simulink model "Equaliser"  (R2021b)
settings: Solver=VariableStepAuto  StartTime=0.0  StopTime=inf  RelTol=1e-3
model workspace (MAT data in the model file):
  D = Simulink.Parameter
  D.DataType = 'auto'
  D.Complexity = 'real'
  D.Dimensions = [0 0]
undefined symbols (not defined in the file): fdesignblkfcn, gcbh
libraries: dspfdesign x2, dspvision x1, dspobslib x1
settings Model: Creator=coren  LastModifiedBy=coren

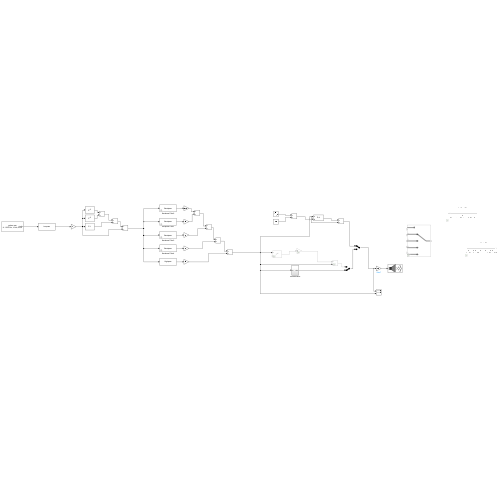
[thumbnail: Simulink's stored preview of the top-level diagram]
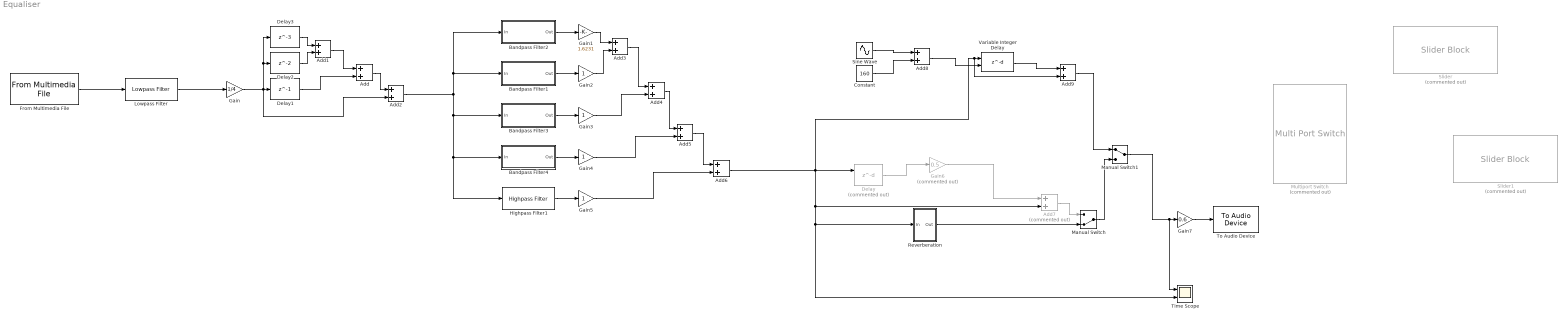
== system Equaliser ==
  Add{,1..6,8..9} (9 alike) : Sum
  Add7 : Sum  Commented=on
  Bandpass Filter1 : Subsystem  DialogController=fdesignblkfcn  InitFcn=fdesignblkfcn(gcbh, {'InitFcn'});  mask(Bandpass Filter){}
      mask help: Design a bandpass filter
      settings: CopyFcn=fdesignblkfcn(gcbh, {'CopyFcn'});
      mask Help: helpview(mapfilelocation('dsp'), 'dspbandpassfilter');
      mask Display: disp('Bandpass');
  Bandpass Filter2 : Subsystem  DialogController=fdesignblkfcn  InitFcn=fdesignblkfcn(gcbh, {'InitFcn'});  mask(Bandpass Filter){}
      mask help: Design a bandpass filter
      settings: CopyFcn=fdesignblkfcn(gcbh, {'CopyFcn'});
      mask Help: helpview(mapfilelocation('dsp'), 'dspbandpassfilter');
      mask Display: disp('Bandpass');
  Bandpass Filter3 : Subsystem  DialogController=fdesignblkfcn  InitFcn=fdesignblkfcn(gcbh, {'InitFcn'});  mask(Bandpass Filter){}
      mask help: Design a bandpass filter
      settings: CopyFcn=fdesignblkfcn(gcbh, {'CopyFcn'});
      mask Help: helpview(mapfilelocation('dsp'), 'dspbandpassfilter');
      mask Display: disp('Bandpass');
  Bandpass Filter4 : Subsystem  DialogController=fdesignblkfcn  InitFcn=fdesignblkfcn(gcbh, {'InitFcn'});  mask(Bandpass Filter){}
      mask help: Design a bandpass filter
      settings: CopyFcn=fdesignblkfcn(gcbh, {'CopyFcn'});
      mask Help: helpview(mapfilelocation('dsp'), 'dspbandpassfilter');
      mask Display: disp('Bandpass');
  Constant : Constant  Value=160
  Delay : Delay  Commented=on  DelayLengthSource=Input port  DelayLength=400  DelayLengthUpperLimit=5000  InputProcessing=Columns as channels (frame based)
      settings: InputPortMap=u0,p1
  Delay1 : Delay  DelayLength=1  DelayLengthUpperLimit=5000  InputProcessing=Columns as channels (frame based)
  Delay2 : Delay  DelayLengthUpperLimit=5000  InputProcessing=Columns as channels (frame based)
  Delay3 : Delay  DelayLength=3  DelayLengthUpperLimit=5000  InputProcessing=Columns as channels (frame based)
  From Multimedia File : dspvision/From Multimedia File  inputFilename=C:\Users\coren\Documents\MATLAB\Traitement Images et Son 3E105\Projet Son\guitare.wav  readRange=[1 Inf]  loop=on  numPlays=inf  outputStreams=Audio only  videoDataType=single  audioDataType=double  inheritSampleTime=on  userDefinedSampleTime=1/30  noAudioOutput=off  isIntensityVideo=off  fourcc=RGB  colorVideoFormat=Separate color signals  outputEOF=off  dataOrg=Column-major  audioFrameSize=1024  computeAudioFrameSize=off  outSamplingMode=Sample based
  Gain : Gain  Gain=1/4
  Gain1 : Gain  Gain=1.6231
  Gain{2..5} (4 alike) : Gain
  Gain6 : Gain  Commented=on  Gain=0.5
  Gain7 : Gain  Gain=0.6
  Highpass Filter1 : dspfdesign/Highpass Filter  FilterType=FIR  DesignForMinimumOrder=on  FilterOrder=50  StopbandFrequency=5412  PassbandFrequency=5512  StopbandAttenuation=80  PassbandRipple=0.1  InheritSampleRate=off  SampleRate=11025  SimulateUsing=Interpreted execution  roundingMode=Floor  coeffsDataTypeStr=fixdt(1,16)
  Lowpass Filter : dspfdesign/Lowpass Filter  FilterType=FIR  DesignForMinimumOrder=on  FilterOrder=50  PassbandFrequency=20e3  StopbandFrequency=21e3  PassbandRipple=0.1  StopbandAttenuation=80  InheritSampleRate=off  SampleRate=44100  SimulateUsing=Interpreted execution  roundingMode=Floor  coeffsDataTypeStr=fixdt(1,16)
  Manual Switch : ManualSwitch  CurrentSetting=0
  Manual Switch1 : ManualSwitch
  Multiport Switch : MultiPortSwitch  Commented=on  DataPortForDefault=Additional data port
  Reverberation : Subsystem
  Sine Wave : Sin  Amplitude=150  Frequency=2*pi*15000  SampleTime=1024
  Slider : SliderBlock  Commented=on  ScaleMin=1  ScaleMax=10
  Slider1 : SliderBlock  Commented=on
  Time Scope : Scope  NumInputPorts=2
  To Audio Device : dspobslib/To Audio Device  deviceName=Default  inheritSampleRate=on  sampleRate=44100  deviceDatatype=Determine from input data type  autoBufferSize=on  bufferSize=4096  queueDuration=1.0  defaultOutputChannelMapping=on  outputChannelMapping=1:2  outputNumUnderrunSamples=off
      settings: SourceProductBaseCode=DS
  Variable Integer Delay : Delay  DelayLengthSource=Input port
      settings: InputPortMap=u0,p1
  wires:
  Add1/1 -> Add/1
  Add/1 -> Add2/1
  Gain/1 -> Delay3/1, Delay2/1, Delay1/1, Add2/2
  Delay1/1 -> Add/2
  Delay3/1 -> Add1/1
  Delay2/1 -> Add1/2
  From Multimedia File/1 -> Lowpass Filter/1
  Lowpass Filter/1 -> Gain/1
  Add2/1 -> Bandpass Filter4/1(In), Highpass Filter1/1, Bandpass Filter3/1(In), Bandpass Filter1/1(In), Bandpass Filter2/1(In)
  Bandpass Filter4/1(Out) -> Gain4/1
  Bandpass Filter3/1(Out) -> Gain3/1
  Bandpass Filter1/1(Out) -> Gain2/1
  Bandpass Filter2/1(Out) -> Gain1/1
  Highpass Filter1/1 -> Gain5/1
  Gain1/1 -> Add3/1
  Gain2/1 -> Add3/2
  Add3/1 -> Add4/1
  Gain3/1 -> Add4/2
  Gain4/1 -> Add5/2
  Add4/1 -> Add5/1
  Add5/1 -> Add6/1
  Gain5/1 -> Add6/2
  Add6/1 -> Delay/1, Reverberation/1(In), Time Scope/2, Add7/2, Add9/2, Variable Integer Delay/1
  Gain7/1 -> To Audio Device/1
  Reverberation/1(Out) -> Manual Switch/2
  Gain6/1 -> Add7/1
  Delay/1 -> Gain6/1
  Add7/1 -> Manual Switch/1
  Sine Wave/1 -> Add8/1
  Constant/1 -> Add8/2
  Add8/1 -> Variable Integer Delay/2
  Variable Integer Delay/1 -> Add9/1
  Add9/1 -> Manual Switch1/1
  Manual Switch/1 -> Manual Switch1/2
  Manual Switch1/1 -> Time Scope/1, Gain7/1

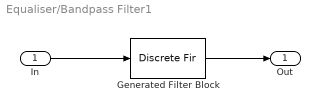
== system Equaliser/Bandpass Filter1 ==
  In : Inport
  Generated Filter Block : DiscreteFir  Tag=BlockMethodSubSystem  Coefficients=[-0.000693909571379187928 -0.000425405216789415098 -0.000413695832590775785 -0.000293308220152275199 -7.99407584597523031e-05 0.000178573895991000645 0.000415310817043652468 0.0005662993121920626 0.000595615969551864001 0.000513535341604299611 0.000380026862224638743 0.000288254097294433952 0.0003318571448728029 0.000564509821100136599 0.00096690260507318541 0.00143323420721916265 0.00178720699380514165 0.00182692258676569476 0.00139041792821636002 0.000420754754861565525 -0.000991002135632512325 -0.00260414815292048284 -0.00407081030418186395 -0.00501960085647781915 -0.00515993188012884522 -0.00437565067436047287 -0.00276952078146972674 -0.000661850949725929696 0.00149127028749933884 0.00321355925068054181 0.00414276410463035316 0.00413602258368764124 0.00331295640237265617 0.00202179386588128987 0.000732640507511793664 -0.000108853346690889819 -0.000224534243761721991 0.000404579888376954699 0.00152732064938441168 0.00270061298957231539 0.00343323600283008089 0.00335144114361827887 0.00233047234221535815 0.000548244255288560288 -0.00156074000496969362 -0.00343884566552071736 -0.00458640135742673441 -0.00472853065314588362 -0.0039122160031066118 -0.00249733114330032147 -0.00104027835781232854 -0.000103130971459907035 -5.64656585280089811e-05 -0.000936083532411734263 -0.00241333092223288163 -0.00388994309728245193 -0.00469402738630428536 -0.0043142160434950852 -0.00259233077662568857 0.000193424009094710753 0.00339082138395853253 0.00616721017050780168 0.00777643024059891056 0.0078101876725220256 0.00634766098253644866 0.00394563943725940742 0.00146492462380448316 -0.000216786734559866148 -0.000511984799328509248 0.000654600292980572394 0.00279123449986311972 0.00497934209024703586 0.00617303100994794334 0.00556313698335482356 0.00288380579442176896 -0.00144802641843132783 -0.00641805186683416708 -0.0107120910056950989 -0.0131336931532712933 -0.0130093885303103063 -0.0104393533624617032 -0.00629940148483808596 -0.00197780459768481407 0.00107953322928640381 0.00187066066525776219 0.000216883947884997859 -0.00312034033064438956 -0.00664241061563812605 -0.00859066469456587489 -0.00755250377124869893 -0.00299898105227922561 0.00443686605542296508 0.0130561229754461387 0.0205623125067658716 0.0247728911195427316 0.0243533998966487843 0.0193269365629533396 0.0111690092664284008 0.002419251801459423 -0.00410223968175413376 -0.00624757933156987102 -0.00335979456960943442 0.00332664944574948516 0.0108803464739269558 0.0154591617694185592 0.013498543073410009 0.00296442363276184888 -0.0157162567775820904 -0.0393701909536459949 -0.0625913374643115999 -0.0789790508199261082 -0.0828062970124469611 -0.0706740065913594312 -0.0426833429939351278 -0.00276356426416210542 0.0419866364388865598 0.0828208613316711723 0.111362364473322831 0.121603070671441812 0.111362364473322831 0.0828208613316711723 0.0419866364388865598 -0.00276356426416210542 -0.0426833429939351278 -0.0706740065913594312 -0.0828062970124469611 -0.0789790508199261082 -0.0625913374643115999 -0.0393701909536459949 -0.0157162567775820904 0.00296442363276184888 0.013498543073410009 0.0154591617694185592 0.0108803464739269558 0.00332664944574948516 -0.00335979456960943442 -0.00624757933156987102 -0.00410223968175413376 0.002419251801459423 0.0111690092664284008 0.0193269365629533396 0.0243533998966487843 0.0247728911195427316 0.0205623125067658716 0.0130561229754461387 0.00443686605542296508 -0.00299898105227922561 -0.00755250377124869893 -0.00859066469456587489 -0.00664241061563812605 -0.00312034033064438956 0.000216883947884997859 0.00187066066525776219 0.00107953322928640381 -0.00197780459768481407 -0.00629940148483808596 -0.0104393533624617032 -0.0130093885303103063 -0.0131336931532712933 -0.0107120910056950989 -0.00641805186683416708 -0.00144802641843132783 0.00288380579442176896 0.00556313698335482356 0.00617303100994794334 0.00497934209024703586 0.00279123449986311972 0.000654600292980572394 -0.000511984799328509248 -0.000216786734559866148 0.00146492462380448316 ...(+1567 chars)]  InputProcessing=Columns as channels (frame based)
  Out : Outport  VectorParamsAs1DForOutWhenUnconnected=off
  wires:
  In/1 -> Generated Filter Block/1
  Generated Filter Block/1 -> Out/1

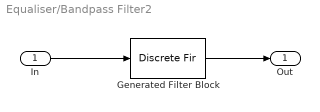
== system Equaliser/Bandpass Filter2 ==
  In : Inport
  Generated Filter Block : DiscreteFir  Tag=BlockMethodSubSystem  Coefficients=[0.000546032994840667642 9.81824061059358155e-05 6.45040991023817416e-05 -5.74861443384752386e-06 -0.000117832939491060041 -0.000276778129251503799 -0.00048534451442133411 -0.00074512730577002838 -0.00105479620135906201 -0.00141128163871280174 -0.00180781941599548524 -0.00223522381366009996 -0.00268072813606996243 -0.0031308894962181321 -0.00357062792007985502 -0.00398046194654954645 -0.00434521049426133971 -0.00464759298163406123 -0.00487285147442745488 -0.00500922923761131823 -0.00504804613494253766 -0.00498578377395045985 -0.00482328674934508553 -0.00456727170133268846 -0.00422911578998918375 -0.00382608968154882342 -0.00337951360651382593 -0.00291460051036349782 -0.00245813368402963278 -0.00203959153412412763 -0.00168591639675533516 -0.00142346016060325171 -0.00127353390090419465 -0.00125299601214107453 -0.00137139139646013275 -0.00163131160844247813 -0.00202649195257598906 -0.00254312338663365434 -0.00315894356694724435 -0.00384528941533711626 -0.00456706042847780831 -0.00528612760841150244 -0.00596203740261236521 -0.00655509379972591018 -0.00702852175422666314 -0.00735107517941025433 -0.00749878886213661833 -0.00745756540728728136 -0.00722353023690021443 -0.00680497191644722534 -0.00622137469449240716 -0.00550388474981680382 -0.00469285273670569554 -0.00383702370069814464 -0.00298999714751253505 -0.00220801267711911216 -0.00154566042851362728 -0.00105371823849921445 -0.000774282085487291234 -0.000739284283384774731 -0.000966454128459402024 -0.00145875246089640091 -0.00220226663916684145 -0.00316713473471645288 -0.0043074496643559744 -0.00556418390706923775 -0.00686716425163908482 -0.00813966234824599864 -0.00930168687357701626 -0.0102758103512429148 -0.0109910791003404902 -0.0113885197234054117 -0.0114248429896392605 -0.0110765337314040896 -0.010341967689480043 -0.00924346773577513874 -0.00782668216256270088 -0.00616003260996819506 -0.00433130016742482981 -0.00244431945108526238 -0.000613015759328147084 0.00104403619470423378 0.00241093572923360873 0.00338097777569463902 0.00386414007960923702 0.0037928443020061155 0.00312821863132733144 0.00186355275492458995 2.77943261183088054e-05 -0.00231418226278283469 -0.00506200298445167157 -0.00808327642235375302 -0.0112179240729523289 -0.0142851906091453571 -0.0170912422199793676 -0.0194387385137691771 -0.0211360651426337198 -0.0220077965184730315 -0.021903836690287809 -0.0207085669212312522 -0.0183480272432440007 -0.0147957998396459102 -0.0100764502562554932 -0.00426704481917435791 0.00250430173715655499 0.0100618442844974659 0.0181885012766653011 0.0266337242964450951 0.0351236702001479495 0.0433723079479413492 0.0510935372602140461 0.0580134400259531419 0.0638822467099486591 0.0684852647569804684 0.0716525430501596117 0.0732662954918938819 0.0732662954918938819 0.0716525430501596117 0.0684852647569804684 0.0638822467099486591 0.0580134400259531419 0.0510935372602140461 0.0433723079479413492 0.0351236702001479495 0.0266337242964450951 0.0181885012766653011 0.0100618442844974659 0.00250430173715655499 -0.00426704481917435791 -0.0100764502562554932 -0.0147957998396459102 -0.0183480272432440007 -0.0207085669212312522 -0.021903836690287809 -0.0220077965184730315 -0.0211360651426337198 -0.0194387385137691771 -0.0170912422199793676 -0.0142851906091453571 -0.0112179240729523289 -0.00808327642235375302 -0.00506200298445167157 -0.00231418226278283469 2.77943261183088054e-05 0.00186355275492458995 0.00312821863132733144 0.0037928443020061155 0.00386414007960923702 0.00338097777569463902 0.00241093572923360873 0.00104403619470423378 -0.000613015759328147084 -0.00244431945108526238 -0.00433130016742482981 -0.00616003260996819506 -0.00782668216256270088 -0.00924346773577513874 -0.010341967689480043 -0.0110765337314040896 -0.0114248429896392605 -0.0113885197234054117 -0.0109910791003404902 -0.0102758103512429148 -0.00930168687357701626 -0.00813966234824599864 -0.00686716425163908482 -0.00556418390706923775 -0.0043074496643559744 -0.00316713473471645288 -0.00220226663916684145 ...(+1493 chars)]  InputProcessing=Columns as channels (frame based)
  Out : Outport  VectorParamsAs1DForOutWhenUnconnected=off
  wires:
  In/1 -> Generated Filter Block/1
  Generated Filter Block/1 -> Out/1

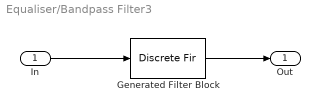
== system Equaliser/Bandpass Filter3 ==
  In : Inport
  Generated Filter Block : DiscreteFir  Tag=BlockMethodSubSystem  Coefficients=[0.000131350560524521486 -0.000937266967500380451 -0.00256900741652817642 -0.00102818462087170422 0.00316408949791832563 0.00651904650434910818 0.00343536326855408162 -0.00410741542831796324 -0.00845523360726441013 -0.00462129394940425861 0.00254283695155502849 0.00510056712529636039 0.00214288568100067011 -0.000150650559183851 0.00133410226775144687 0.00254030166370671547 -0.000299683656292623298 -0.00400774796457640213 -0.00356395727332833433 -0.000193926004261525377 0.000916985498850044108 -0.000718654941960008469 -0.000550200452261146431 0.00266006518921109956 0.00425663804763064865 0.00148491275416990243 -0.00170003999621341924 -0.00122051769406387122 0.000388743359936229627 -0.00119842961664260871 -0.00405222326434478107 -0.00295298151853342532 0.00143896218278335422 0.00323354219419490782 0.00107040711900155037 0.000147007206974752899 0.00276456130692947361 0.00387543811251532836 -0.000130809218363982916 -0.00449396417268808565 -0.0035672917712431646 -0.000217851865779361396 -0.000636739898116213876 -0.00328075750330997186 -0.00147942836575721279 0.00431946451143210876 0.00624007128714557362 0.00198266795074408244 -0.00122768076865015468 0.000866270420036095246 0.00216766487461260557 -0.00265840328034424016 -0.00770108045322803227 -0.00503216181841400784 0.0015945278507455017 0.00274621662872646466 -0.000674638907950892396 0.000582761038408930007 0.00696310660048309309 0.00801880402480105448 0.000234406656934269697 -0.00598105695058128058 -0.00335743715890193502 0.000157234057829705047 -0.00405465362410570556 -0.00903180302608506437 -0.00364551583843327138 0.00710220630356327414 0.00897192323939476587 0.00213019200883200494 0.000455369381337614003 0.00664346213961594309 0.00666450805965165295 -0.00517722898368941538 -0.0139498142563244075 -0.00795960461190261571 0.00134760250290166589 -0.000850094254849310298 -0.00651629296734033362 0.0010699539547963132 0.015784939023625412 0.0160224873493072656 0.00110703690059309906 -0.00641683797422956496 0.000849717940210375534 0.00232106346978039378 -0.0130100711661859467 -0.0232674924215618278 -0.00892156083911045845 0.0117471611231694337 0.0112214628485626765 -0.000450559202197350992 0.00646119274741744579 0.025837392310702232 0.02103956184551245 -0.0112810485144069304 -0.0289522245739111464 -0.0126478990505932698 -0.000155784669315973642 -0.0200472432595015689 -0.0343174991949406483 0.00139741958831116498 0.0523430950488528654 0.0489818930429722285 0.00416956370667097113 0.000687361622517842011 0.0446300163269386235 0.0270565741143310515 -0.102662570693366206 -0.204222748594201559 -0.10209086898986415 0.149411144086683018 0.284819232874632899 0.149411144086683018 -0.10209086898986415 -0.204222748594201559 -0.102662570693366206 0.0270565741143310515 0.0446300163269386235 0.000687361622517842011 0.00416956370667097113 0.0489818930429722285 0.0523430950488528654 0.00139741958831116498 -0.0343174991949406483 -0.0200472432595015689 -0.000155784669315973642 -0.0126478990505932698 -0.0289522245739111464 -0.0112810485144069304 0.02103956184551245 0.025837392310702232 0.00646119274741744579 -0.000450559202197350992 0.0112214628485626765 0.0117471611231694337 -0.00892156083911045845 -0.0232674924215618278 -0.0130100711661859467 0.00232106346978039378 0.000849717940210375534 -0.00641683797422956496 0.00110703690059309906 0.0160224873493072656 0.015784939023625412 0.0010699539547963132 -0.00651629296734033362 -0.000850094254849310298 0.00134760250290166589 -0.00795960461190261571 -0.0139498142563244075 -0.00517722898368941538 0.00666450805965165295 0.00664346213961594309 0.000455369381337614003 0.00213019200883200494 0.00897192323939476587 0.00710220630356327414 -0.00364551583843327138 -0.00903180302608506437 -0.00405465362410570556 0.000157234057829705047 -0.00335743715890193502 -0.00598105695058128058 0.000234406656934269697 0.00801880402480105448 0.00696310660048309309 0.000582761038408930007 -0.000674638907950892396 0.00274621662872646466 0.0015945278507455017 -0.00503216181841400784 ...(+1257 chars)]  InputProcessing=Columns as channels (frame based)
  Out : Outport  VectorParamsAs1DForOutWhenUnconnected=off
  wires:
  In/1 -> Generated Filter Block/1
  Generated Filter Block/1 -> Out/1

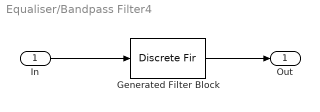
== system Equaliser/Bandpass Filter4 ==
  In : Inport
  Generated Filter Block : DiscreteFir  Tag=BlockMethodSubSystem  Coefficients=[-0.00236772825052023426 0.00420756839900255242 -0.000416134564502849166 -0.00744294413557698535 0.00994996518054239512 -0.0044809618507501486 0.000379099854429861916 -0.00293832603710013959 0.00508573702881190241 -0.00226062192737525687 0.000619525138638663052 -0.00321284079631067735 0.00403593332942066719 -0.00153439452963973475 0.00154072649114648358 -0.00401651751658666824 0.00344731299298835746 -0.00141415316517396004 0.00279519250265993207 -0.00456583967234471585 0.00283470693203389948 -0.00183669639409400902 0.00412779264720996002 -0.00460252987069179314 0.00232352674988080049 -0.00281197242918601034 0.00520986740134935129 -0.00411785739833225948 0.00221130169462715846 -0.00419140970453804086 0.00571655574087062603 -0.00334607198288396123 0.00274976119918578623 -0.00561920314315103066 0.00546661492029465804 -0.00269735629919436865 0.0039664635532504957 -0.00661943294037768172 0.00456815855935271704 -0.00263708363116410506 0.00559654882591072156 -0.00678068607295957259 0.00341756920941239852 -0.00344161515849552907 0.00710167155343855837 -0.0059721575668550634 0.0026208979591728996 -0.00504627176062706802 0.00785936866611653719 -0.00445663902646663973 0.00272939233721228823 -0.00697261528257425017 0.00743460168062340734 -0.00287617857020253716 0.00398182958860117311 -0.00845850628813425015 0.00582588655087745884 -0.00202942639368603166 0.0061069972488034148 -0.00874887293043626231 0.00356872167678565526 -0.00253159060369509718 0.00833450057237781691 -0.00745410503136317761 0.00160920043984312229 -0.00448140866034118547 0.00963944989714857897 -0.00482036191578511138 0.000952605897557793528 -0.00728835273018945112 0.00916314006828538967 -0.00176383403792973871 0.00221070360818341775 -0.00979706594839176333 0.00666104819801471848 0.000400092156922223212 0.00521377620241716359 -0.0106799941059954155 0.00276178209739949337 0.000459564443301996328 0.00891848961468255132 -0.0090230374367872828 -0.00110931359474069464 -0.00209863942680708904 0.011658142632185297 -0.00484228530974228737 -0.00317001252228602025 -0.00670122072674603653 0.0117517395542713066 0.00068489746037998431 -0.00199075111971921655 -0.0116564556044269768 0.0082391493947127567 0.00542846349022522035 0.00279853268540050486 -0.0145945933108735885 0.00148834580900902651 0.00694411628221485149 0.0100755126853474437 -0.0132621251679409975 -0.00659034716549475319 0.00335517909945406631 0.0172476534309157284 -0.00638900436361726498 -0.0128324253445982316 -0.00585669088260752733 0.0207737932430752045 0.00563642854792477822 -0.0134267425141898281 -0.0194148528410483211 0.016710986459258205 0.0207121395308006023 -0.00429993439577626337 -0.0345252246103173385 0.000553549123804408425 0.0354390940875586383 0.0208393407038131966 -0.0474991929595444326 -0.0397526160797662051 0.046163333060289781 0.0960103079139505294 -0.0549891398421562053 -0.310927471893762852 0.550082266413271959 -0.310927471893762852 -0.0549891398421562053 0.0960103079139505294 0.046163333060289781 -0.0397526160797662051 -0.0474991929595444326 0.0208393407038131966 0.0354390940875586383 0.000553549123804408425 -0.0345252246103173385 -0.00429993439577626337 0.0207121395308006023 0.016710986459258205 -0.0194148528410483211 -0.0134267425141898281 0.00563642854792477822 0.0207737932430752045 -0.00585669088260752733 -0.0128324253445982316 -0.00638900436361726498 0.0172476534309157284 0.00335517909945406631 -0.00659034716549475319 -0.0132621251679409975 0.0100755126853474437 0.00694411628221485149 0.00148834580900902651 -0.0145945933108735885 0.00279853268540050486 0.00542846349022522035 0.0082391493947127567 -0.0116564556044269768 -0.00199075111971921655 0.00068489746037998431 0.0117517395542713066 -0.00670122072674603653 -0.00317001252228602025 -0.00484228530974228737 0.011658142632185297 -0.00209863942680708904 -0.00110931359474069464 -0.0090230374367872828 0.00891848961468255132 0.000459564443301996328 0.00276178209739949337 -0.0106799941059954155 0.00521377620241716359 0.000400092156922223212 ...(+1762 chars)]  InputProcessing=Columns as channels (frame based)
  Out : Outport  VectorParamsAs1DForOutWhenUnconnected=off
  wires:
  In/1 -> Generated Filter Block/1
  Generated Filter Block/1 -> Out/1

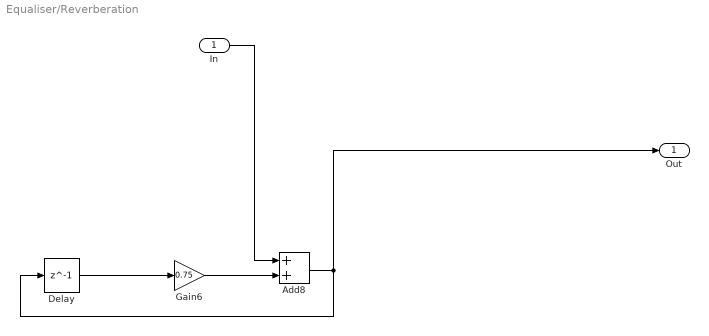
== system Equaliser/Reverberation ==
  In : Inport
  Add8 : Sum
  Delay : Delay  DelayLength=1
  Gain6 : Gain  Gain=0.75
  Out : Outport
  wires:
  Delay/1 -> Gain6/1
  Add8/1 -> Out/1, Delay/1
  Gain6/1 -> Add8/2
  In/1 -> Add8/1
